simulink model "zaj3simulink"  (R2020b)
settings: Solver=odeN  StartTime=0.0  StopTime=2000.0  RelTol=1e-3
values from neighbouring files (symbols this model uses):
  cv1 = ro*cp*v1    (= 108540)    [zaj1.m]
  cv2 = ro*cp*v2    (= 36180)    [zaj1.m]
  dqg = 1000    [zaj1.m]
  dTzew = 0    [zaj1.m]
  k = 1.75/dqg    (= 0.00175)    [zaj1.m]
  Ks0 = (Ks2*(T2N-TzewN))/(T1N-T2N)    (= 903.225806452)    [zaj1.m]
  Ks1 = 3*Ks2    (= 387.096774194)    [zaj1.m]
  Ks2 = QgN/(3*(T1N-TzewN)+T2N-TzewN)    (= 129.032258065)    [zaj1.m]
  QgN = 20000    [zaj1.m]
  steptime = 100    [zaj1.m]
  T = 300    [zaj1.m]
  T1N = 20    [zaj1.m]
  T2N = 15    [zaj1.m]
  T_0 = 10    [zaj1.m]
  tw10d = [cv1*cv2 cv1*Ks0+cv1*Ks2+Ks1*cv2+Ks0*cv2 Ks0*Ks1+Ks2*Ks0+Ks1*Ks2]    [zaj1.m]
  tw1intinit = T1N    (= 20)    [zaj1.m]
  tw2intinit = T2N    (= 15)    [zaj1.m]
  TzewN = -20    [zaj1.m]
settings Model: Creator=bilin  LastModifiedBy=bilin
settings SolverCC: MaxConsecutiveZCs=10000

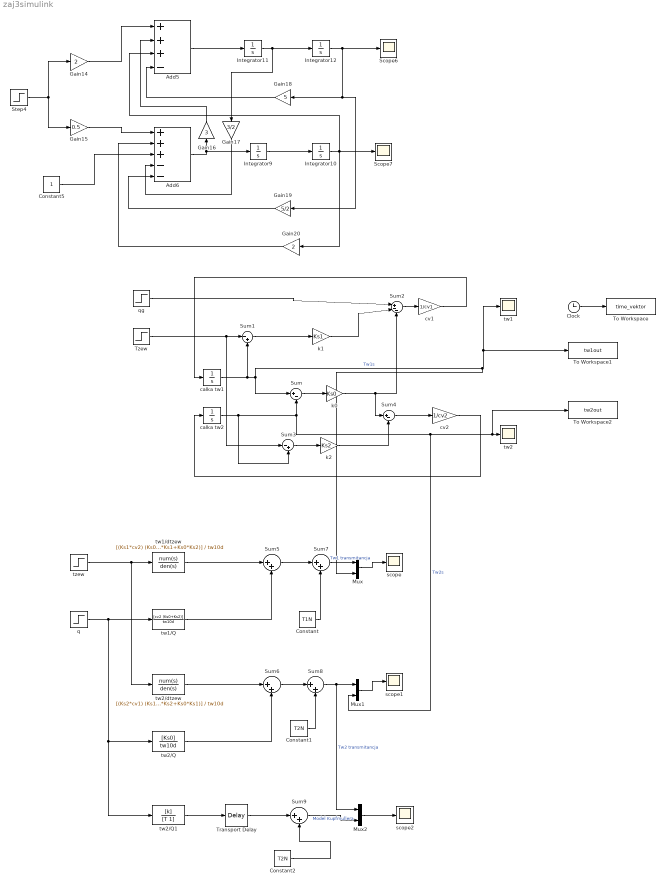
== system zaj3simulink ==
  Add5 : Sum  Inputs=+++-
  Add6 : Sum  Inputs=+++--
  Clock : Clock
  Constant : Constant  Value=T1N
  Constant1 : Constant  Value=T2N
  Constant2 : Constant  Value=T2N
  Constant5 : Constant
  Gain14 : Gain  Gain=2
  Gain15 : Gain  Gain=0.5
  Gain16 : Gain  Gain=3
  Gain17 : Gain  Gain=3/2
  Gain18 : Gain  Gain=5
  Gain19 : Gain  Gain=5/2
  Gain20 : Gain  Gain=2
  Integrator{9..12} (4 alike) : Integrator
  Mux : Mux  Inputs=2
  Mux1 : Mux  Inputs=2
  Mux2 : Mux  Inputs=2
  Scope6 : Scope
  Scope7 : Scope
  Step4 : Step  Time=10  After=5  SampleTime=0
  Sum : Sum  Inputs=|+-
  Sum1 : Sum  Inputs=|-+
  Sum2 : Sum  Inputs=|+--
  Sum3 : Sum  Inputs=|-+
  Sum4 : Sum  Inputs=|+-
  Sum{5..9} (5 alike) : Sum  Inputs=|++
  To Workspace : ToWorkspace  VariableName=time_vektor  SampleTime=-1
  To Workspace1 : ToWorkspace  VariableName=tw1out  SampleTime=-1
  To Workspace2 : ToWorkspace  VariableName=tw2out  SampleTime=-1
  Transport Delay : TransportDelay  DelayTime=T_0
  Tzew : Step  Time=steptime  Before=TzewN  After=TzewN+dTzew  SampleTime=0
  calka tw1 : Integrator  InitialCondition=tw1intinit
  calka tw2 : Integrator  InitialCondition=tw2intinit
  cv1 : Gain  Gain=1/cv1
  cv2 : Gain  Gain=1/cv2
  k0 : Gain  Gain=Ks0
  k1 : Gain  Gain=Ks1
  k2 : Gain  Gain=Ks2
  q : Step  Time=steptime  After=dqg  SampleTime=0
  qg : Step  Time=steptime  Before=QgN  After=QgN+dqg  SampleTime=0
  scope : Scope
  scope1 : Scope
  scope2 : Scope
  tw1 : Scope
  tw1/Q : TransferFcn  Numerator=[cv2 (Ks0+Ks2)]  Denominator=tw10d
  tw1/dtzew : TransferFcn  Numerator=[(Ks1*cv2) (Ks0*Ks1+Ks2*Ks1+Ks0*Ks2)]  Denominator=tw10d
  tw2 : Scope
  tw2/Q : TransferFcn  Numerator=[Ks0]  Denominator=tw10d
  tw2/Q1 : TransferFcn  Numerator=[k]  Denominator=[T 1]
  tw2/dtzew : TransferFcn  Numerator=[(Ks2*cv1) (Ks1*Ks2+Ks0*Ks2+Ks0*Ks1)]  Denominator=tw10d
  tzew : Step  Time=steptime  After=dTzew  SampleTime=0
  wires:
  Gain20/1 -> Add6/2
  Integrator10/1 -> Scope7/1, Gain20/1, Add5/3
  Constant5/1 -> Add6/3
  Gain19/1 -> Add6/5
  Gain17/1 -> Add6/4
  Gain18/1 -> Add5/4
  Integrator12/1 -> Gain18/1, Gain19/1, Scope6/1
  Integrator11/1 -> Integrator12/1, Gain17/1
  Add5/1 -> Integrator11/1
  Integrator9/1 -> Integrator10/1
  Gain16/1 -> Add5/2
  Add6/1 -> Gain16/1, Integrator9/1
  Gain15/1 -> Add6/1
  Gain14/1 -> Add5/1
  Step4/1 -> Gain14/1, Gain15/1
  calka tw1/1 -> Sum1/2, Mux/2, To Workspace1/1, tw1/1, Sum/1  "Tw1s"
  calka tw2/1 -> Sum3/2, To Workspace2/1, tw2/1, Mux1/2, Sum/2  "Tw2s"
  Sum/1 -> k0/1
  Tzew/1 -> Sum3/1, Sum1/1
  Sum1/1 -> k1/1
  qg/1 -> Sum2/1
  k1/1 -> Sum2/2
  k0/1 -> Sum4/1, Sum2/3
  Sum2/1 -> cv1/1
  Sum3/1 -> k2/1
  k2/1 -> Sum4/2
  Sum4/1 -> cv2/1
  cv2/1 -> calka tw2/1
  cv1/1 -> calka tw1/1
  Clock/1 -> To Workspace/1
  tzew/1 -> tw2/dtzew/1, tw1/dtzew/1
  tw1/dtzew/1 -> Sum5/1
  tw1/Q/1 -> Sum5/2
  q/1 -> tw2/Q/1, tw2/Q1/1, tw1/Q/1
  tw2/Q/1 -> Sum6/2
  tw2/dtzew/1 -> Sum6/1
  Sum5/1 -> Sum7/1
  Constant/1 -> Sum7/2
  Sum6/1 -> Sum8/1
  Constant1/1 -> Sum8/2
  Sum7/1 -> Mux/1  "Tw1 transmitancja"
  Mux/1 -> scope/1
  Mux1/1 -> scope1/1
  Sum8/1 -> Mux1/1, Mux2/1  "Tw2 transmitancja"
  tw2/Q1/1 -> Transport Delay/1
  Constant2/1 -> Sum9/2
  Transport Delay/1 -> Sum9/1
  Mux2/1 -> scope2/1
  Sum9/1 -> Mux2/2  "Model Kupfmullera"
